simulink model "lineFollowing"  (R2023a)
settings: Solver=FixedStepDiscrete  StartTime=0.0  StopTime=30  FixedStep=0.01  RelTol=1e-3
values from neighbouring files (symbols this model uses):
  axleLength = 0.136    [robotParameters.m]
  maxV = (160/30)*pi*wheelR    (= 0.519409985394)    [robotParameters.m]
  ticksPerRot = 20    [robotParameters.m]
  wheelR = 0.031    [robotParameters.m]
undefined symbols (not defined in the file or in its folder): InputPWM, WheelSpeed
libraries: mobileRoboticsTrainingLib x10, slpidlib x1
settings Model: Creator=Boitumelo  LastModifiedBy=friso
settings DebuggingCC: UnconnectedInputMsg=warning  UnconnectedOutputMsg=warning  UnconnectedLineMsg=warning
settings ModelReferenceCC: EnableRefExpFcnMdlSchedulingChecks=on
settings RTWCC: DLArmComputeVersion=19.05

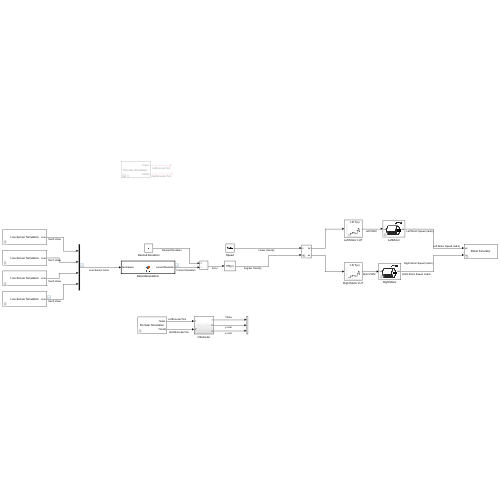
[thumbnail: Simulink's stored preview of the top-level diagram]
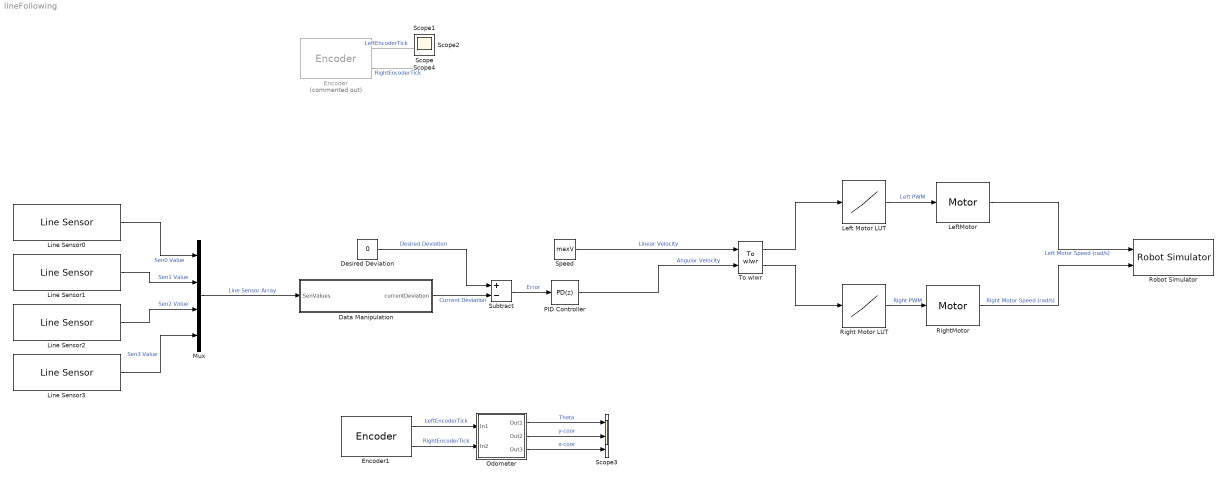
== system lineFollowing ==
  Data Manipulation : MATLAB Function  TreatAsAtomicUnit=on
  Desired Deviation : Constant  Value=0
  Encoder : mobileRoboticsTrainingLib/Encoder  Commented=on  axleLength=axleLength  wheelR=wheelR  ticksPerRot=ticksPerRot
      settings: SourceProductName=Mobile Robotics Training Library
  Encoder1 : mobileRoboticsTrainingLib/Encoder  axleLength=axleLength  wheelR=wheelR  ticksPerRot=ticksPerRot
      settings: SourceProductName=Mobile Robotics Training Library
  Left Motor LUT : Lookup_n-D  NumberOfTableDimensions=1  BreakpointsForDimension1=WheelSpeed  Table=InputPWM  InterpMethod=Nearest  ExtrapMethod=Clip  InternalRulePriority=Speed  RndMeth=Simplest
  LeftMotor : mobileRoboticsTrainingLib/Motor  motorPlant=wheelMotorModel  sensorType=Speed
      settings: SourceProductName=Mobile Robotics Training Library
  Line Sensor0 : mobileRoboticsTrainingLib/Line Sensor  mapVariable=mapForSim  envVal=2800  lineVal=2900  sensOff=[0.0643 0.0353]
      settings: SourceProductName=Mobile Robotics Training Library
  Line Sensor1 : mobileRoboticsTrainingLib/Line Sensor  mapVariable=mapForSim  envVal=2800  lineVal=2900  sensOff=[0.0675 0.005]
      settings: SourceProductName=Mobile Robotics Training Library
  Line Sensor2 : mobileRoboticsTrainingLib/Line Sensor  mapVariable=mapForSim  envVal=2800  lineVal=2900  sensOff=[0.0643 -0.0353]
      settings: SourceProductName=Mobile Robotics Training Library
  Line Sensor3 : mobileRoboticsTrainingLib/Line Sensor  mapVariable=mapForSim  envVal=2800  lineVal=2900  sensOff=[0.0675 -0.005]
      settings: SourceProductName=Mobile Robotics Training Library
  Mux : Mux
  Odometer : Subsystem
  PID Controller : slpidlib/PID Controller  Controller=PD  Form=Parallel  TimeDomain=Discrete-time  UseExternalTs=off  SampleTime=-1  IntegratorMethod=Forward Euler  FilterMethod=Forward Euler  ControllerParametersSource=internal  P=0.2  I=1  UseKiTs=off  D=1e-5  N=100  UseFilter=on  TunerSelectOption=Frequency Response Based  InitialConditionSource=internal  InitialConditionForIntegrator=0  InitialConditionForFilter=0  DifferentiatorICPrevScaledInput=0  ExternalReset=none  TrackingMode=off  Kt=1  LimitOutput=off  SatLimitsSource=internal  UpperSaturationLimit=inf  LowerSaturationLimit=-inf  LinearizeAsGain=on  AntiWindupMode=none  Kb=1  LimitIntegrator=off  UpperIntegratorSaturationLimit=inf  LowerIntegratorSaturationLimit=-inf  POutMin=[]  POutMax=[]  IOutMin=[]  IOutMax=[]  DOutMin=[]  DOutMax=[]  NOutMin=[]  NOutMax=[]  SumOutMin=[]  SumOutMax=[]  SaturationOutMin=[]  SaturationOutMax=[]  PParamMin=[]  PParamMax=[]  IParamMin=[]  IParamMax=[]  DParamMin=[]  DParamMax=[]  NParamMin=[]  NParamMax=[]  KbParamMin=[]  KbParamMax=[]  KtParamMin=[]  KtParamMax=[]  KbOutMin=[]  KbOutMax=[]  KtOutMin=[]  KtOutMax=[]  IntegratorOutMin=[]  IntegratorOutMax=[]  FilterOutMin=[]  FilterOutMax=[]  SumI1OutMin=[]  SumI1OutMax=[]  SumI2OutMin=[]  SumI2OutMax=[]  SumI3OutMin=[]  SumI3OutMax=[]  SumI4OutMin=[]  SumI4OutMax=[]  SumDOutMin=[]  SumDOutMax=[]  DifferentiatorOutMin=[]  DifferentiatorOutMax=[]  FilterDiffOutCoefMin=[]  FilterDiffOutCoefMax=[]  ReciprocalOutMin=[]  ReciprocalOutMax=[]  SumDenOutMin=[]  SumDenOutMax=[]  SumNumOutMin=[]  SumNumOutMax=[]  DivideOutMin=[]  DivideOutMax=[]  UdiffTsProdOutMin=[]  UdiffTsProdOutMax=[]  NTsProdOutMin=[]  NTsProdOutMax=[]  UintegralTsProdOutMin=[]  UintegralTsProdOutMax=[]  UngainTsProdOutMin=[]  UngainTsProdOutMax=[]  ClampingZeroOutDataTypeStr=Inherit: Inherit via back propagation  ClampingZeroOutMin=[]  ClampingZeroOutMax=[]  FilterDenConstantOutDataTypeStr=Inherit: Inherit via back propagation  FilterDenConstantOutMin=[]  FilterDenConstantOutMax=[]  PCopyOutDataTypeStr=Inherit: Inherit via back propagation  PCopyOutMin=[]  PCopyOutMax=[]  NCopyOutDataTypeStr=Inherit: Inherit via back propagation  NCopyOutMin=[]  NCopyOutMax=[]  IntegratorContinuousStateAttributes=''  IntegratorStateMustResolveToSignalObject=off  IntegratorRTWStateStorageClass=Auto  FilterContinuousStateAttributes=''  FilterStateMustResolveToSignalObject=off  FilterRTWStateStorageClass=Auto  ParallelPVariant=InternalParameters  IdealPVariant=Disabled  IVariant=Disabled  DVariant=InternalParameters  IntegratorVariant=Disabled  SatVariant=Disabled  AWVariant=Disabled  PCopyVariant=Disabled  TRVariant=Disabled  FdbkBlocksVariant=Forward  IdealPFdbkVariant=Disabled  SatFdbkVariant=Disabled  DerivativeFilterVariant=ForwardEulerFilter  NVariant=InternalParameters  NCopyVariant=Disabled  FilterICVariant=InternalICsFilter  IntegratorICVariant=Disabled  ExternalResetVariant=Disabled  TRSumVariant=Passthrough  SumFdbkVariant=Disabled  SumVariant=Sum_PD  TsampFilterVariant=InternalTs  TsampNgainVariant=Passthrough  TsampIntegralVariant=Disabled_SignalSpec  ExternalSaturationOutDataTypeStr=Inherit: Same as second input
  Right Motor LUT : Lookup_n-D  NumberOfTableDimensions=1  BreakpointsForDimension1=WheelSpeed  Table=InputPWM  InterpMethod=Nearest  ExtrapMethod=Clip  InternalRulePriority=Speed  RndMeth=Simplest
  RightMotor : mobileRoboticsTrainingLib/Motor  motorPlant=wheelMotorModel  sensorType=Speed
      settings: SourceProductName=Mobile Robotics Training Library
  Robot Simulator : mobileRoboticsTrainingLib/Robot Simulator  Priority=99  mapVar=mapForSim  startX=xInitial  startY=yInitial  startTheta=90  axleLength=axleLength  wheelR=wheelR
  Scope3 : Scope  NumInputPorts=3
  Speed : Constant  Value=maxV
  Subtract : Sum  Inputs=+-
  To wlwr : mobileRoboticsTrainingLib/To wlwr  axleLength=0.1  wheelR=0.05
  Scope{,1..2,4} (4 alike) : Scope
  wires:
  Right Motor LUT/1 -> RightMotor/1  "Right PWM"
  Left Motor LUT/1 -> LeftMotor/1  "Left PWM"
  Encoder/1 -> ?  "LeftEncoderTick"
  Encoder/2 -> ?  "RightEncoderTick"
  To wlwr/1 -> Left Motor LUT/1
  To wlwr/2 -> Right Motor LUT/1
  RightMotor/1 -> Robot Simulator/2  "Right Motor Speed (rad/s)"
  LeftMotor/1 -> Robot Simulator/1  "Left Motor Speed (rad/s)"
  Desired Deviation/1 -> Subtract/1  "Desired Deviation"
  Subtract/1 -> PID Controller/1  "Error"
  Speed/1 -> To wlwr/1  "Linear Velocity"
  PID Controller/1 -> To wlwr/2  "Angular Velocity"
  Data Manipulation/1(currentDeviation) -> Subtract/2  "Current Deviation"
  Mux/1 -> Data Manipulation/1(SenValues)  "Line Sensor Array"
  Line Sensor0/1 -> Mux/1  "Sen0 Value"
  Line Sensor1/1 -> Mux/2  "Sen1 Value"
  Line Sensor2/1 -> Mux/3  "Sen2 Value"
  Line Sensor3/1 -> Mux/4  "Sen3 Value"
  Odometer/3(Out3) -> Scope3/3  "x-coor"
  Encoder1/1 -> Odometer/1(In1)  "LeftEncoderTick"
  Encoder1/2 -> Odometer/2(In2)  "RightEncoderTick"
  Odometer/2(Out2) -> Scope3/2  "y-coor"
  Odometer/1(Out1) -> Scope3/1  "Theta"

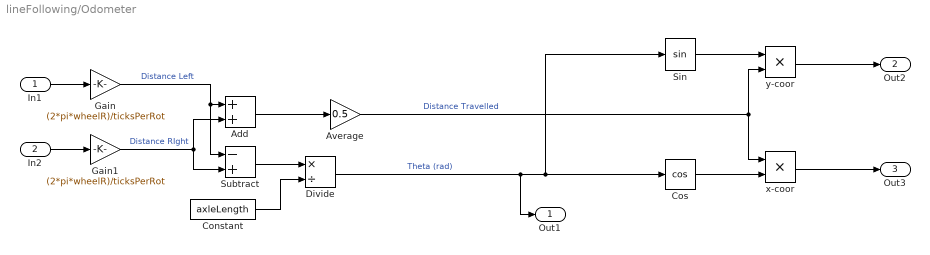
== system lineFollowing/Odometer ==
  In1 : Inport
  In2 : Inport  Port=2
  Add : Sum
  Average : Gain  Gain=0.5
  Constant : Constant  Value=axleLength
  Cos : Trigonometry  Operator=cos  OutputSignalType=real
  Divide : Product  Inputs=*/
  Gain : Gain  Gain=(2*pi*wheelR)/ticksPerRot
  Gain1 : Gain  Gain=(2*pi*wheelR)/ticksPerRot
  Sin : Trigonometry  OutputSignalType=real
  Subtract : Sum  Inputs=-+
  x-coor : Product
  y-coor : Product
  Out1 : Outport
  Out2 : Outport  Port=2
  Out3 : Outport  Port=3
  wires:
  x-coor/1 -> Out3/1
  Divide/1 -> Out1/1, Sin/1, Cos/1  "Theta (rad)"
  Gain/1 -> Subtract/1, Add/1  "Distance Left"
  In1/1 -> Gain/1
  Cos/1 -> x-coor/2
  Subtract/1 -> Divide/1
  Add/1 -> Average/1
  Average/1 -> x-coor/1, y-coor/2  "Distance Travelled"
  Gain1/1 -> Add/2, Subtract/2  "Distance RIght"
  Sin/1 -> y-coor/1
  In2/1 -> Gain1/1
  Constant/1 -> Divide/2
  y-coor/1 -> Out2/1

== matlab function lineFollowing/Data Manipulation ==
  data: SenValues input; currentDeviation output
function currentDeviation = fcn(SenValues)
totalZero = 0; % Initialize number of sensors not detecting lines
for i=1:1:size(SenValues, 1)
    if (SenValues(i) == 2800)
        totalZero = totalZero + 1;  % Determine number of sensors not detecting lines
    end
end

if totalZero == 0
    currentDeviation = 0; % Divide by 0 case 
else
    currentDeviation = ((SenValues(1)*-2)+(SenValues(2)*-1)+(SenValues(3)*1)+(SenValues(4)*2))/totalZero; % Normalized representation of deviation
end
